simulink library "UAVdesign_net"  (Simulink 7.7)
settings: Solver=ode45  SolverMode=SingleTasking  StartTime=0.0  StopTime=10.0  RelTol=1e-3
undefined symbols (not defined in the file or in its folder): alpha_IERA_IELA_IELA, R_IERA_RA_RA
libraries: UAVdesign_net x75, simulink x13
(part 1 of 8)
settings Model: Creator=Emanuel  LastModifiedBy=Emanuel

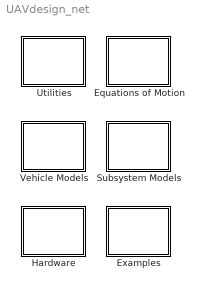
== system UAVdesign_net ==
  Equations of Motion : Subsystem
      mask Display: disp('Equations of\nMotion')
  Examples : Subsystem
      settings: OpenFcn=UAVdesign_net_examples
      mask Display: disp('Examples')
  Hardware : Subsystem
      mask Display: disp('Hardware\nI/O')
  Subsystem Models : Subsystem
      mask Display: disp('Subsystem\nModels')
  Utilities : Subsystem
      mask Display: disp('Utilities')
  Vehicle Models : Subsystem
      mask Display: disp('Vehicle\nModels')

== system UAVdesign_net/Equations of Motion ==
  6DoF Equations of Motion : Subsystem  TreatAsAtomicUnit=on  mask(6DoFEoM){}
      mask help: 6DoF using Euler angles.
      mask Display:
      | port_label('input',1,'V_b(xyz)','texmode','on');
      | port_label('input',2,'\omega_b(xyz)','texmode','on');
      | port_label('input',3,'R_e(NED)','texmode','on');
      | port_label('input',4,'\alpha_e(\phi,\theta,\psi)','texmode','on');
      | port_label('input',5,'F_{ext}(xyz)','texmode','on');
      | port_label('input',6,'M_{ext}(xyz)','texmode','on');
      | port_label('input',7,'m','texmode','on');
      | port_label('input',8,'In_b','texmode','on');
      | port_label('output',1,'V_bdot(xyz)','texmode','on');
      | port_label('output',2,'\omega_bdot(xyz)','texmode','on');
      | port_label('output',3,'R_edot(NED)','texmode','on');
      | port_label('output',4,'\alpha_edot(\phi,\theta,\psi)','texmode','on');
  6DoF Equations of Motion (Quaternions) : Subsystem  TreatAsAtomicUnit=on  mask(6DoFEoMQuaternions){}
      mask help: 6DoF using quaternions.
      mask Display:
      | port_label('input',1,'V_b (xyz)','texmode','on');
      | port_label('input',2,'\omega_b (xyz)','texmode','on');
      | port_label('input',3,'R_e (NED)','texmode','on');
      | port_label('input',4,'q (a_0 a)','texmode','on');
      | port_label('input',5,'F_{ext} (xyz)','texmode','on');
      | port_label('input',6,'M_{ext} (xyz)','texmode','on');
      | port_label('input',7,'m','texmode','on');
      | port_label('input',8,'In_b','texmode','on');
      | port_label('output',1,'V_b^\bullet (xyz)','texmode','on');
      | port_label('output',2,'\omega_b^\bullet (xyz)','texmode','on');
      | port_label('output',3,'R_e^\bullet (NED)','texmode','on');
      | port_label('output',4,'q^\bullet (a_0 a)','texmode','on');

== system UAVdesign_net/Examples ==

== system UAVdesign_net/Hardware ==
  Generic Comm : Subsystem  mask(GenericComm){devicetype=UDP port, com_port='COM4', baud=115200, host_name='192.168.1.10', remote_port=60500, local_port=60500, timeout=1, rx_size=54, handshake=on, sample_time=-1}
      mask prompts: devicetype "Device Type"; com_port "COM port (string between single quotes, e.g. 'COM4' or 'ttyACM0')"; baud "Baud Rate"; host_name "Host Name (string between single quotes, e.g. '192.168.1.10')"; remote_port "Transmit to UDP port"; local_port "Listen on UDP port"; timeout "Timeout (sec)"; rx_size "RX vector size (bytes)"; handshake "Enable handshaking (for the Basestation)"; sample_time "Sample Time"
      mask help:
      | Generic communication block.
      | Allows communication to take place using either a serial port or UDP packets.
      mask init:
      | UAVdesign_net_generic_comm_callback(gcb, 0, 0, com_port, host_name, remote_port, local_port)
      mask StyleString: popup(COM port|UDP port),edit,edit,edit,edit,edit,edit,edit,checkbox,edit
      mask CallbackString: UAVdesign_net_generic_comm_callback(gcb, 1, 0)|||||||||
      mask Display: text(0.1, 0.7, '192.168.1.10'); text(0.1, 0.3, 'L:60500  R:60500')
  Generic Comm Example : Subsystem  mask(GenericCommExample){devicetype=COM port, com_port='COM4', baud=115200, host_name='192.168.1.10', remote_port=60500, local_port=60500, timeout=1}
      mask prompts: devicetype "Device Type"; com_port "COM port"; baud "Baud Rate"; host_name "Host Name"; remote_port "Remote UDP port"; local_port "Local UDP port"; timeout "Timeout (sec)"
      mask help: Example of how to transfer parameters to a Generic Comm block behind a mask.
      mask init:
      | start = 0;
      | a=get_param([gcb '/Generic Comm'], 'MaskStyles');
      | b=get_param(gcb, 'MaskStyles');
      | b{start+1}=a{1};
      | set_param(gcb, 'MaskStyles', b);
      | 
      | a=get_param(gcb, 'MaskValues');
      | b=get_param([gcb '/Generic Comm'], 'MaskValues');
      | b{1}=a{start+1};
      | set_param([gcb '/Generic Comm'], 'MaskValues', b);
      mask StyleString: popup(COM port|UDP port),edit,edit,edit,edit,edit,edit
      mask CallbackString:
      | start = 0;
      | UAVdesign_net_generic_comm_callback(gcb, 1, start)||||||
  GigE Camera : S-Function  FunctionName=gigecomm  Parameters=host,img_size,format,raw_data,soft_trig,timeout,st  EnableBusSupport=off  mask(GigE_Camera){host='192.168.2.20', img_size=[640 480 1], format=Rgb24, raw_data=off, soft_trig=off, timeout=1, st=1/20}
      mask prompts: host "Remote Host (string between single quotes, e.g. '192.168.1.10')"; img_size "Image size [x y N]"; format "Pixel format"; raw_data "Dump raw data"; soft_trig "Software Trigger"; timeout "Timeout (sec)"; st "Sample Time"
      mask help: GigE camera
      mask StyleString: edit,edit,popup(Mono8|Mono16|Bayer8|Bayer16|Rgb24|Rgb48|Yuv411|Yuv422|Yuv444),checkbox,checkbox,edit,edit
      mask Display:
      | text(0.1, 0.7, host)
      | text(0.1, 0.3, [num2str(img_size(1)) 'x' num2str(img_size(2))])
  Serial Port : S-Function  FunctionName=serialcomm  Parameters=port,baud_rate,timeout,tx_enable,rx_enable,receive,num_packets_overrun,num_packets_received,st  EnableBusSupport=off  mask(SerialPort){port='COM4', baud_rate=115200, timeout=1, tx_enable=on, rx_enable=on, receive=46, num_packets_overrun=off, num_packets_received=off, st=-1}
      mask prompts: port "COM port (string between single quotes, e.g. 'COM4' or 'ttyACM0')"; baud_rate "Baud Rate"; timeout "Timeout (sec)"; tx_enable "Enable TX"; rx_enable "Enable RX"; receive "RX vector size (bytes)"; num_packets_overrun "Leave one packet in the RX buffer if more are received"; num_packets_received "Output the number of packets received"; st "Sample Time"
      mask help: Timeout: If positive, the transfers are blocking for the specified amount, and if no data arrives then an error will be generated. If zero, the available data in the buffer (if any) will be transferred. If negative, blocking transfers will occur and no timeout will be used.
      mask Display: disp(port);
  Simulation Rate : S-Function  FunctionName=simulationrate  Parameters=SimSampleTime  EnableBusSupport=off  mask(SimulationRate){SimSampleTime=1/20}
      mask prompts: SimSampleTime "Simulation Sample Time"
      mask help: Slows down the simulation to a rate close to real-time.
      mask Display: disp('Sim Rate')
  Simulation Time : S-Function  FunctionName=display_time_sfun  Parameters=sample_time  EnableBusSupport=off  mask(DisplayTime){sample_time=-1}
      mask prompts: sample_time "Input Sample Time"
      mask help: This block displays the simulation time in the Matlab workspace for debugging purposes.
      mask Display: port_label('Output', 1, 'Time');
  Thread Priority : S-Function  FunctionName=threadpriority  Parameters=PolicySimWin,PolicyExtWin,PolicySimLinux,PolicyExtLinux,PrioritySimWin,PriorityExtWin,PrioritySimLinux,PriorityExtLinux  EnableBusSupport=off  mask(ThreadPriority){PolicySimWin=Normal, PolicyExtWin=Normal, PolicySimLinux=SCHED_OTHER, PolicyExtLinux=SCHED_OTHER, PrioritySimWin=0, PriorityExtWin=0, PrioritySimLinux=0, PriorityExtLinux=-6}
      mask prompts: PolicySimWin "Thread policy (Windows, Simulation)"; PolicyExtWin "Thread policy (Windows, External)"; PolicySimLinux "Thread policy (Linux, Simulation)"; PolicyExtLinux "Thread policy (Linux, External)"; PrioritySimWin "Thread priority (Windows, Simulation)"; PriorityExtWin "Thread priority (Windows, External)"; PrioritySimLinux "Thread priority (Linux, Simulation)"; PriorityExtLinux "Thread priority (Linux, External)"
      mask help:
      | For Linux, the priorities specify:
      |   - the nice value for the SCHED_OTHER policy
      |     (-20 for maximum priority, 19 for minimum, 0 for default)
      |   - the real-time priority for the other two options
      |     (1 for minimum priority, 98 for maximum priority).
      mask StyleString: popup(Normal|Real Time),popup(Normal|Real Time),popup(SCHED_OTHER|SCHED_FIFO|SCHED_RR),popup(SCHED_OTHER|SCHED_FIFO|SCHED_RR),edit,edit,edit,edit
      mask Display: disp('Priority')
  To Multimedia File : S-Function  FunctionName=tomultimediafile  Parameters=format, file_name, force_rate, frame_rate, sample_time  EnableBusSupport=off  mask(ToMMFile){format=Raw, file_name='test.bin', force_rate=off, frame_rate=25, sample_time=-1}
      mask prompts: format "File Format"; file_name "File Name (between commas, e.g. 'test.avi')"; force_rate "Force a specific frame rate in the header"; frame_rate "Frame Rate (to be included in the file header)"; sample_time "Sample Time"
      mask help: Saves the data to a file in different formats.
      mask init:
      | maskval = get_param(gcb, 'MaskValues');
      | visibility = get_param(gcb, 'MaskVisibilities');
      | if strcmp(maskval{3}, 'on')
      |     visibility{4} = 'on';
      | else
      |     visibility{4} = 'off';
      | end
      | set_param(gcb, 'MaskVisibilities', visibility);
      mask StyleString: popup(Raw|AVI|WAV),edit,checkbox,edit,edit
      mask CallbackString:
      | ||maskval = get_param(gcb, 'MaskValues');
      | visibility = get_param(gcb, 'MaskVisibilities');
      | if strcmp(maskval{3}, 'on')
      |     visibility{4} = 'on';
      | else
      |     visibility{4} = 'off';
      | end
      | set_param(gcb, 'MaskVisibilities', visibility);
      | clear maskval visibility
      | ||
      mask Display: disp(file_name)
  Type Conversion : S-Function  FunctionName=datatypeconv_sfun  Parameters=indim, intype, outdim, outtype, signextend  EnableBusSupport=off  mask(TypeConversion){indim=4, intype=uint8, outdim=1, outtype=unsigned double, signextend=off}
      mask prompts: indim "Input Dimension"; intype "Input Type"; outdim "Output Dimension"; outtype "Output Type"; signextend "Sign Extend the Input"
      mask help: Converts between data types while keeping the binary representation.
      mask init:
      | tstr = {'dbl' 'sgl' 'int8' 'uint8' 'int16' 'uint16' 'int32' 'uint32' 'bool' 'udbl' 'usgl'};
      | dispstr = [tstr{intype} ' \rightarrow ' tstr{outtype}];
      mask StyleString: edit,popup(double|single|int8|uint8|int16|uint16|int32|uint32|boolean),edit,popup(double|single|int8|uint8|int16|uint16|int32|uint32|boolean|unsigned double|unsigned single),checkbox
      mask Display: disp(dispstr, 'texmode', 'on')
  UDP : S-Function  FunctionName=udpcomm  Parameters=host,local_port,remote_port,timeout,tx_enable,rx_enable,receive,num_packets_overrun,num_packets_received,handshake,st  EnableBusSupport=off  mask(UDPPort){host='192.168.2.20', remote_port=60500, local_port=60500, timeout=1, tx_enable=on, rx_enable=on, receive=46, num_packets_overrun=off, num_packets_received=off, handshake=on, st=-1}
      mask prompts: host "Remote Host (string between single quotes, e.g. '192.168.1.10')"; remote_port "Transmit to UDP port"; local_port "Listen on UDP port"; timeout "Timeout (sec)"; tx_enable "Enable TX"; rx_enable "Enable RX"; receive "Receive vector size (bytes)"; num_packets_overrun "Leave one packet in the RX buffer if more are received"; num_packets_received "Output the number of packets received"; handshake "Enable handshaking (for the Basestation)"; st "Sample Time"
      mask help: Timeout: If positive, the transfers are blocking for the specified amount, and if no data arrives then an error will be generated. If zero, the available data in the buffer (if any) will be transferred. If negative, blocking transfers will occur and no timeout will be used.
      mask Display:
      | text(0.1, 0.7, host)
      | text(0.1, 0.3, ['L:' num2str(local_port) '  R:' num2str(remote_port)])

== system UAVdesign_net/Subsystem Models ==
  DC Motor (Electrical) : Subsystem  TreatAsAtomicUnit=on
      mask Type: HelicopterMotor
      mask Description: DC Motor model.
      mask Display:
      | port_label('input', 1, 'Parameters', 'texmode', 'on')
      | port_label('input', 2, 'Voltage', 'texmode', 'on')
      | port_label('input', 3, '\Omega_{rotor-stator}', 'texmode', 'on')
      | 
      | port_label('output', 1, '\tau_{motor}', 'texmode', 'on')
  Fin : Subsystem  TreatAsAtomicUnit=on
      mask Type: HelicopterFinModel
      mask Description: Fin model.
      mask Display:
      | port_label('input', 1, 'Parameters', 'texmode', 'on')
      | port_label('input', 2, 'Environment', 'texmode', 'on')
      | port_label('input', 3, 'R_{IELA-B|B}', 'texmode', 'on')
      | port_label('input', 4, 'T_{IERA-IELA}', 'texmode', 'on')
      | port_label('input', 5, 'V_{B-E|B}', 'texmode', 'on')
      | port_label('input', 6, '\omega_{B-E|B}', 'texmode', 'on')
      | port_label('input', 7, 'V_{W|B}', 'texmode', 'on')
      | port_label('input', 8, '\omega_{W|B}', 'texmode', 'on')
      | 
      | port_label('output', 1, 'FM_{B}', 'texmode', 'on')
      | port_label('output', 2, 'FM_{IELA}', 'texmode', 'on')
      | port_label('output', 3, 'd_{IELA}', 'texmode', 'on')
      | port_label('output', 4, 'V \omega_{A|IELA}', 'texmode', 'on')
  Fuselage : Subsystem  TreatAsAtomicUnit=on
      mask Type: HelicopterFuselageModel
      mask Description: Fuselage model.
      mask Display:
      | port_label('input', 1, 'Parameters', 'texmode', 'on')
      | port_label('input', 2, 'Environment', 'texmode', 'on')
      | port_label('input', 3, 'R_{IELA-B|B}', 'texmode', 'on')
      | port_label('input', 4, 'T_{IERA-IELA}', 'texmode', 'on')
      | port_label('input', 5, 'V_{B-E|B}', 'texmode', 'on')
      | port_label('input', 6, '\omega_{B-E|B}', 'texmode', 'on')
      | port_label('input', 7, 'V_{W|B}', 'texmode', 'on')
      | port_label('input', 8, '\omega_{W|B}', 'texmode', 'on')
      | 
      | port_label('output', 1, 'FM_{B}', 'texmode', 'on')
      | port_label('output', 2, 'FM_{IELA}', 'texmode', 'on')
      | port_label('output', 3, 'd_{IELA}', 'texmode', 'on')
      | port_label('output', 4, 'V \omega_{A|IELA}', 'texmode', 'on')
  Helicopter Parameters : Subsystem  mask(HelicopterParameters){}
      mask help:
      | Parameters for a helicopter.
      | Geometry, rotors, fuselage, fins.
      mask init:
      | set_param(gcb, 'LinkStatus', 'none');
      settings: OpenFcn=gui_HelicopterParameters( 'Block', [get_param(gcb, 'Parent') '/' get_param(gcb, 'Name')]);
      mask Display:
      | port_label('output', 1, 'Parameters')
      | port_label('output', 2, 'Geometry')
  Helicopter Rotor : Subsystem  TreatAsAtomicUnit=on
      mask Type: HelicopterRotorModel
      mask Description: Model of a helicopter rotor
      mask Display:
      | port_label('input', 1, 'Parameters', 'texmode', 'on')
      | port_label('input', 2, 'Environment', 'texmode', 'on')
      | port_label('input', 3, 'R_{IELA-B|B}', 'texmode', 'on')
      | port_label('input', 4, 'T_{IERA-IELA}', 'texmode', 'on')
      | port_label('input', 5, 'V_{B-E|B}', 'texmode', 'on')
      | port_label('input', 6, '\omega_{B-E|B}', 'texmode', 'on')
      | port_label('input', 7, 'V^\bullet_{B-E|B}', 'texmode', 'on')
      | port_label('input', 8, '\omega^\bullet_{B-E|B}', 'texmode', 'on')
      | port_label('input', 9, 'V_{W|B}', 'texmode', 'on')
      | port_label('input', 10, '\omega_{W|B}', 'texmode', 'on')
      | port_label('input', 11, '\Omega_{rotor}', 'texmode', 'on')
      | port_label('input', 12, '\Omega^\bullet_{rotor}', 'texmode', 'on')
      | port_label('input', 13, 'controls_{IERA}', 'texmode', 'on')
      | port_label('input', 14, 'tilt^\bullet_{nac}', 'texmode', 'on')
      | port_label('input', 15, 'flap_{(k-1)|IERA}', 'texmode', 'on')
      | port_label('input', 16, 'd_{k-1|IELA}', 'texmode', 'on')
      | port_label('input', 17, 'bt_{k-1}', 'texmode', 'on')
      | port_label('input', 18, 'eps0_{k-1}', 'texmode', 'on')
      | 
      | port_label('output', 1, 'FM_{B}', 'texmode', 'on')
      | port_label('output', 2, 'FM_{IELA}', 'texmode', 'on')
      | port_label('output', 3, 'flap^\bullet_{IERA}', 'texmode', 'on')
      | port_label('output', 4, 'd_{k|IELA}', 'texmode', 'on')
      | port_label('output', 5, 'bt_{k}', 'texmode', 'on')
      | port_label('output', 6, 'eps0_{k}', 'texmode', 'on')
      | port_label('output', 7, 'flap_{k|IERA}', 'texmode', 'on')
      | port_label('output', 8, 'T Q', 'texmode', 'on')
      | port_label('output', 9, 'V \omega_{A|IELA}', 'texmode', 'on')
  Propeller : Subsystem  TreatAsAtomicUnit=on
      mask Type: HelicopterPropellerModel
      mask Description: Model of a rigid propeller
      mask Display:
      | port_label('input', 1, 'Parameters', 'texmode', 'on')
      | port_label('input', 2, 'Environment', 'texmode', 'on')
      | port_label('input', 3, 'R_{IELA-B|B}', 'texmode', 'on')
      | port_label('input', 4, 'T_{IERA-IELA}', 'texmode', 'on')
      | port_label('input', 5, 'V_{B-E|B}', 'texmode', 'on')
      | port_label('input', 6, '\omega_{B-E|B}', 'texmode', 'on')
      | port_label('input', 7, 'V_{W|B}', 'texmode', 'on')
      | port_label('input', 8, '\omega_{W|B}', 'texmode', 'on')
      | port_label('input', 9, '\Omega_{rotor}', 'texmode', 'on')
      | port_label('input', 10, '\tau_{motor}', 'texmode', 'on')
      | port_label('input', 11, 'pitch', 'texmode', 'on')
      | port_label('input', 12, 'd_{k-1|IELA}', 'texmode', 'on')
      | port_label('input', 13, 'bt_{k-1}', 'texmode', 'on')
      | port_label('input', 14, 'eps0_{k-1}', 'texmode', 'on')
      | 
      | port_label('output', 1, 'FM_{B}', 'texmode', 'on')
      | port_label('output', 2, 'FM_{IELA}', 'texmode', 'on')
      | port_label('output', 3, 'd_{k|IELA}', 'texmode', 'on')
      | port_label('output', 4, 'bt_{k}', 'texmode', 'on')
      | port_label('output', 5, 'eps0_{k}', 'texmode', 'on')
      | port_label('output', 6, 'T Q', 'texmode', 'on')
      | port_label('output', 7, 'V \omega_{A|IELA}', 'texmode', 'on')
  Propeller Rotation Dynamics : Subsystem  TreatAsAtomicUnit=on
      mask Type: HelicopterPropellerRotDynamics
      mask Description: The rotation dynamics for a rigid propeller
      mask Display:
      | port_label('input', 1, 'Parameters', 'texmode', 'on')
      | port_label('input', 2, 'T_{IERA-IELA}', 'texmode', 'on')
      | port_label('input', 3, '\tau_{prop} (Q)', 'texmode', 'on')
      | port_label('input', 4, '\tau_{motor}', 'texmode', 'on')
      | port_label('input', 5, '\omega_{B-E|B}', 'texmode', 'on')
      | port_label('input', 6, '\omega^\bullet_{B-E|B}', 'texmode', 'on')
      | port_label('input', 7, '\Omega_{rotor}', 'texmode', 'on')
      | 
      | port_label('output', 1, '\Omega^\bullet_{rotor}', 'texmode', 'on')
  QuadRotor Parameters : Subsystem  InitFcn=|  mask(HelicopterParameters){}
      | bus_PropellerParameters;    
      | bus_ElectricMotorParameters;
      | bus_GeometryParameters;     
      | bus_FuselageParameters;
      mask help:
      | Parameters for a helicopter.
      | Geometry, rotors, fuselage, fins.
      mask init:
      | set_param(gcb, 'LinkStatus', 'none');
      settings: OpenFcn=gui_QuadRotorParameters( 'Block', [get_param(gcb, 'Parent') '/' get_param(gcb, 'Name')]);
      mask Display:
      | port_label('output', 1, 'Parameters')
      | port_label('output', 2, 'Geometry')
  Wing : Subsystem  TreatAsAtomicUnit=on
      mask Type: HelicopterWingModel
      mask Description: Wing model.
      mask Display:
      | port_label('input', 1, 'Parameters', 'texmode', 'on')
      | port_label('input', 2, 'Environment', 'texmode', 'on')
      | port_label('input', 3, 'R_{IELA-B|B}', 'texmode', 'on')
      | port_label('input', 4, 'T_{IERA-IELA}', 'texmode', 'on')
      | port_label('input', 5, 'V_{B-E|B}', 'texmode', 'on')
      | port_label('input', 6, '\omega_{B-E|B}', 'texmode', 'on')
      | port_label('input', 7, 'V_{W|B}', 'texmode', 'on')
      | port_label('input', 8, '\omega_{W|B}', 'texmode', 'on')
      | 
      | port_label('output', 1, 'FM_{B}', 'texmode', 'on')
      | port_label('output', 2, 'FM_{IELA}', 'texmode', 'on')
      | port_label('output', 3, 'd_{IELA}', 'texmode', 'on')
      | port_label('output', 4, 'V \omega_{A|IELA}', 'texmode', 'on')

== system UAVdesign_net/Utilities ==
  Axes : Subsystem
      mask Display: disp('Axes\nTransf.')
  Continuous : Subsystem
      mask Display: disp('Continuous')
  Kalman Filter : Subsystem
      mask Display: disp('Kalman\nFilter')
  Math : Subsystem
      mask Display: disp('Math\nOperations')
  Numeric Perturbation : Subsystem
      mask Display: disp('Numeric\nPerturbation')
  Unit Conversion : Subsystem
      mask Display: disp('Unit\nConversions')

== system UAVdesign_net/Vehicle Models ==
  Helicopter Model : Subsystem  InitFcn=|  TreatAsAtomicUnit=on
      | bus_RotorParameters;
      | bus_FuselageParameters;
      | bus_FinParameters;
      | bus_GeometryParameters;
      | bus_Environment;
      mask Type: HelicopterModel
      mask Description:
      | Model of a helicopter.
      | Derived from "Introduction to Helicopter and Tiltrotor Flight Simulation" by Mark Dreier.
      mask Display:
      | port_label('input', 1, 'Parameters (bus)', 'texmode', 'on')
      | port_label('input', 2, 'Geometry (bus)', 'texmode', 'on')
      | port_label('input', 3, 'Environment (bus)', 'texmode', 'on')
      | port_label('input', 4, 'controls', 'texmode', 'on')
      | port_label('input', 5, '\Omega_{rotor} MR', 'texmode', 'on')
      | port_label('input', 6, '\Omega_{rotor} TR', 'texmode', 'on')
      | port_label('input', 7, 'xc', 'texmode', 'on')
      | port_label('input', 8, 'xc^\bullet_{k-1}', 'texmode', 'on')
      | port_label('input', 9, 'xd_{k-1}', 'texmode', 'on')
      | 
      | port_label('output', 1, 'xc^\bullet', 'texmode', 'on')
      | port_label('output', 2, 'xd_{k}', 'texmode', 'on')
      | port_label('output', 3, 'flap_{k}', 'texmode', 'on')
      | port_label('output', 4, '[info] FM_{CG}', 'texmode', 'on')
      | port_label('output', 5, '[info] FM_{IELA}', 'texmode', 'on')
      | port_label('output', 6, '[info] d_{IELA}', 'texmode', 'on')
      | port_label('output', 7, '[info] V \omega_{W|IELA}', 'texmode', 'on')
      | port_label('output', 8, '[info] V \omega_{A|IELA}', 'texmode', 'on')
      | port_label('output', 9, '[info] TQ rotors', 'texmode', 'on')
  Helicopter Parameters : Subsystem  mask(HelicopterParameters){}
      mask help:
      | Parameters for a helicopter.
      | Geometry, rotors, fuselage, fins.
      mask init:
      | set_param(gcb, 'LinkStatus', 'none');
      settings: OpenFcn=gui_HelicopterParameters( 'Block', [get_param(gcb, 'Parent') '/' get_param(gcb, 'Name')]);
      mask Display:
      | port_label('output', 1, 'Parameters')
      | port_label('output', 2, 'Geometry')
  Quad-Rotor Model (Momentum) : Subsystem  InitFcn=|  TreatAsAtomicUnit=on
      | bus_PropellerParameters;    
      | bus_ElectricMotorParameters;
      | bus_FuselageParameters;     
      | bus_GeometryParameters;     
      | bus_Environment;
      mask Type: HelicopterModel
      mask Description: Model of a quadrotor
      mask Display:
      | port_label('input', 1, 'Parameters (bus)', 'texmode', 'on')
      | port_label('input', 2, 'Geometry (bus)', 'texmode', 'on')
      | port_label('input', 3, 'Environment (bus)', 'texmode', 'on')
      | port_label('input', 4, 'V_{mot}', 'texmode', 'on')
      | port_label('input', 5, 'Wind_e', 'texmode', 'on')
      | port_label('input', 6, 'xc', 'texmode', 'on')
      | port_label('input', 7, 'xd_{k-1}', 'texmode', 'on')
      | 
      | port_label('output', 1, 'info (bus)', 'texmode', 'on')
      | port_label('output', 2, 'xc^\bullet', 'texmode', 'on')
      | port_label('output', 3, 'xd_{k}', 'texmode', 'on')
  QuadRotor Parameters : Subsystem  InitFcn=|  mask(HelicopterParameters){}
      | bus_PropellerParameters;    
      | bus_ElectricMotorParameters;
      | bus_GeometryParameters;     
      | bus_FuselageParameters;
      mask help:
      | Parameters for a helicopter.
      | Geometry, rotors, fuselage, fins.
      mask init:
      | set_param(gcb, 'LinkStatus', 'none');
      settings: OpenFcn=gui_QuadRotorParameters( 'Block', [get_param(gcb, 'Parent') '/' get_param(gcb, 'Name')]);
      mask Display:
      | port_label('output', 1, 'Parameters')
      | port_label('output', 2, 'Geometry')
  wires:
  QuadRotor Parameters/1(Parameters) -> Quad-Rotor Model (Momentum)/1(ParametersBus)
  QuadRotor Parameters/2(Geometry) -> Quad-Rotor Model (Momentum)/2(GeometryBus)
  Helicopter Parameters/1(Parameters) -> Helicopter Model/1(ParametersBus)
  Helicopter Parameters/2(Geometry) -> Helicopter Model/2(GeometryBus)

== system UAVdesign_net/Equations of Motion/6DoF Equations of Motion ==
  Body velocities (V_b) : Inport  PortDimensions=3
  Angular velocities (omega_b) : Inport  Port=2  PortDimensions=3
  Inertial positions (R_e) : Inport  Port=3  PortDimensions=3
  Euler angles(Alpha_e) : Inport  Port=4  PortDimensions=3
  Forces (F_xyz) : Inport  Port=5  PortDimensions=3
  Moments (M_xyz) : Inport  Port=6  PortDimensions=3
  Mass (m) : Inport  Port=7  PortDimensions=1
  Inertia matrix (In_b) : Inport  Port=8  PortDimensions=[3 3]
  3x3 Cross Product : UAVdesign_net/Utilities/Math/3x3 Cross Product  SystemSampleTime=-1
  3x3 Cross Product1 : UAVdesign_net/Utilities/Math/3x3 Cross Product  SystemSampleTime=-1
  Euler Rotation Matrix from Body to Earth : UAVdesign_net/Utilities/Axes/Euler Rotation Matrix from Body to Earth  SystemSampleTime=-1
  Invert  3x3 Matrix1 : UAVdesign_net/Utilities/Math/Invert  3x3 Matrix  SystemSampleTime=-1
  Math Function : Math  Operator=reciprocal  SaturateOnIntegerOverflow=on
  Product{,1,4..5} (4 alike) : Product  Multiplication=Matrix(*)  RndMeth=Zero
  Product2 : Product  RndMeth=Zero
  Product3 : Product  RndMeth=Zero
  Rotation Matrix for angular rates Body to Earth : UAVdesign_net/Utilities/Axes/Rotation Matrix for angular rates Body to Earth  SystemSampleTime=-1
  Sum : Sum  Inputs=|+-
  Sum1 : Sum  Inputs=|+-
  Terminator : Terminator
  Body accelerations (V_b_dot) : Outport
  Angular accelerations (omega_b_dot) : Outport  Port=2
  Inertial velocities (R_e_dot) : Outport  Port=3
  Euler velocities (alpha_e_dot) : Outport  Port=4
  wires:
  Rotation Matrix for angular rates Body to Earth/1 -> Product1/1
  Inertial positions (R_e)/1 -> Terminator/1
  Product4/1 -> Angular accelerations (omega_b_dot)/1
  Product5/1 -> 3x3 Cross Product1/2
  3x3 Cross Product1/1 -> Sum1/2
  Moments (M_xyz)/1 -> Sum1/1
  Sum1/1 -> Product4/2
  Invert  3x3 Matrix1/1 -> Product4/1
  Inertia matrix (In_b)/1 -> Invert  3x3 Matrix1/1, Product5/1
  Product2/1 -> Body accelerations (V_b_dot)/1
  Product3/1 -> 3x3 Cross Product/2
  3x3 Cross Product/1 -> Sum/2
  Forces (F_xyz)/1 -> Sum/1
  Sum/1 -> Product2/2
  Math Function/1 -> Product2/1
  Mass (m)/1 -> Math Function/1, Product3/1
  Product1/1 -> Euler velocities (alpha_e_dot)/1
  Angular velocities (omega_b)/1 -> 3x3 Cross Product/1, 3x3 Cross Product1/1, Product5/2, Product1/2
  Product/1 -> Inertial velocities (R_e_dot)/1
  Body velocities (V_b)/1 -> Product3/2, Product/2
  Euler Rotation Matrix from Body to Earth/1 -> Product/1
  Euler angles(Alpha_e)/1 -> Rotation Matrix for angular rates Body to Earth/1, Euler Rotation Matrix from Body to Earth/1

== system UAVdesign_net/Equations of Motion/6DoF Equations of Motion (Quaternions) ==
  V_b : Inport  PortDimensions=3
  omega_b : Inport  Port=2  PortDimensions=3
  R_e : Inport  Port=3  PortDimensions=3
  q : Inport  Port=4  PortDimensions=4
  F_xyz : Inport  Port=5  PortDimensions=3
  M_xyz : Inport  Port=6  PortDimensions=3
  Mass : Inport  Port=7  PortDimensions=1
  Inertia matrix (In_b) : Inport  Port=8  PortDimensions=[3 3]
  3x3 Cross Product : UAVdesign_net/Utilities/Math/3x3 Cross Product  SystemSampleTime=-1
  3x3 Cross Product1 : UAVdesign_net/Utilities/Math/3x3 Cross Product  SystemSampleTime=-1
  Divide : Product  Inputs=*/
  Gain : Gain  Gain=1/2
  Invert  3x3 Matrix : UAVdesign_net/Utilities/Math/Invert  3x3 Matrix  SystemSampleTime=-1
  Product : Product  Multiplication=Matrix(*)  RndMeth=Zero
  Product1 : Product  Multiplication=Matrix(*)  RndMeth=Zero
  Quaternion Multiplication : UAVdesign_net/Utilities/Math/Quaternion Multiplication  SystemSampleTime=-1
  Quaternion Rotation (E<B) : UAVdesign_net/Utilities/Math/Quaternion Rotation (E<B)  SystemSampleTime=-1
  Sum : Sum  Inputs=|-+
  Sum1 : Sum  Inputs=+-|
  Terminator : Terminator
  Vector to Quaternion : UAVdesign_net/Utilities/Math/Vector to Quaternion  SystemSampleTime=-1
  V_b_dot : Outport
  omega_b_dot : Outport  Port=2
  R_e_dot : Outport  Port=3
  q_dot : Outport  Port=4
  wires:
  Quaternion Multiplication/1 -> q_dot/1
  Vector to Quaternion/1 -> Quaternion Multiplication/2
  Gain/1 -> Quaternion Multiplication/1
  R_e/1 -> Terminator/1
  Quaternion Rotation (E<B)/1 -> R_e_dot/1
  q/1 -> Gain/1, Quaternion Rotation (E<B)/1
  Product/1 -> omega_b_dot/1
  3x3 Cross Product1/1 -> Sum1/2
  M_xyz/1 -> Sum1/1
  Product1/1 -> 3x3 Cross Product1/2
  Invert  3x3 Matrix/1 -> Product/1
  Sum1/1 -> Product/2
  Inertia matrix (In_b)/1 -> Product1/1, Invert  3x3 Matrix/1
  Sum/1 -> V_b_dot/1
  Divide/1 -> Sum/2
  3x3 Cross Product/1 -> Sum/1
  V_b/1 -> Quaternion Rotation (E<B)/2, 3x3 Cross Product/2
  omega_b/1 -> Vector to Quaternion/1, Product1/2, 3x3 Cross Product1/1, 3x3 Cross Product/1
  Mass/1 -> Divide/2
  F_xyz/1 -> Divide/1

== system UAVdesign_net/Hardware/Generic Comm ==
  TX : Inport
  UDP : UAVdesign_net/Hardware/UDP  host=host_name  remote_port=remote_port  local_port=local_port  timeout=timeout  tx_enable=on  rx_enable=on  receive=rx_size  num_packets_overrun=off  num_packets_received=on  handshake=on  st=sample_time
  RX : Outport
  num_rx_packets : Outport  Port=2
  wires:
  TX/1 -> UDP/1
  UDP/1 -> RX/1
  UDP/2 -> num_rx_packets/1

== system UAVdesign_net/Hardware/Generic Comm Example ==
  In1 : Inport
  Generic Comm : UAVdesign_net/Hardware/Generic Comm  SystemSampleTime=-1  devicetype=COM port  com_port=com_port  baud=baud  host_name=host_name  remote_port=remote_port  local_port=local_port  timeout=timeout  rx_size=54  handshake=on  sample_time=-1
  Out1 : Outport
  Out2 : Outport  Port=2

== system UAVdesign_net/Subsystem Models/DC Motor (Electrical) ==
  Parameters : Inport
  V : Inport  Port=2  PortDimensions=1
  omega : Inport  Port=3  PortDimensions=1
  Bus Selector : BusSelector  OutputSignals=R,Kv,Kt
  Divide : Product  Inputs=*/
  Product : Product  RndMeth=Zero
  Product1 : Product  Inputs=**/  RndMeth=Zero
  Sum : Sum  Inputs=|+-
  tork : Outport  PortDimensions=1
  wires:
  Parameters/1 -> Bus Selector/1
  Bus Selector/1 -> Divide/2  "<R>"
  Bus Selector/2 -> Product1/3  "<Kv>"
  Bus Selector/3 -> Product/1, Product1/1  "<Kt>"
  V/1 -> Product/2
  Product/1 -> Sum/1
  Product1/1 -> Sum/2
  Sum/1 -> Divide/1
  Divide/1 -> tork/1
  omega/1 -> Product1/2

== system UAVdesign_net/Subsystem Models/Fin ==
  Parameters : Inport  OutDataTypeStr=Bus: FinParameters
  Environment : Inport  Port=2  OutDataTypeStr=Bus: Environment
  R_IELA_B_B : Inport  Port=3  PortDimensions=3
  T_IERA_IELA : Inport  Port=4  PortDimensions=[3 3]
  V_B_E_B : Inport  Port=5  PortDimensions=3
  omega_B_E_B : Inport  Port=6  PortDimensions=3
  V_W : Inport  Port=7  PortDimensions=3
  omega_W : Inport  Port=8  PortDimensions=3
  CG to IELA : Subsystem
      mask Display:
      | port_label('input', 1, 'R_{IELA-B|B}', 'texmode', 'on')
      | port_label('input', 2, 'V_{B-E|B}', 'texmode', 'on')
      | port_label('input', 3, '\omega_{B-E|B}', 'texmode', 'on')
      | port_label('output', 1, 'V_{IELA-E|IELA}', 'texmode', 'on')
      | port_label('output', 2, '\omega_{IELA-E|IELA}', 'texmode', 'on')
  Fin Model (IERA) : Subsystem
      mask Display:
      | port_label('input', 1, 'Parameters', 'texmode', 'on')
      | port_label('input', 2, 'Environment', 'texmode', 'on')
      | port_label('input', 3, 'V_{A}', 'texmode', 'on')
      | port_label('input', 4, '\omega_{A}', 'texmode', 'on')
      | port_label('input', 5, 'V_{W}', 'texmode', 'on')
      | port_label('input', 6, '\omega_{W}', 'texmode', 'on')
      | port_label('input', 7, 'control', 'texmode', 'on')
      | 
      | port_label('output', 1, 'FM_{I}', 'texmode', 'on')
      | port_label('output', 2, 'FM_{A}', 'texmode', 'on')
      | port_label('output', 3, 'd_{k}', 'texmode', 'on')
  IELA to CG : Subsystem
      mask Display:
      | port_label('input', 1, 'R_{IELA-B|B}', 'texmode', 'on')
      | port_label('input', 2, 'FM_{IELA}', 'texmode', 'on')
      | port_label('output', 1, 'FM_{B}', 'texmode', 'on')
  IELA to IERA : Subsystem
      mask Display:
      | port_label('input', 1, 'T_{IERA-IELA}', 'texmode', 'on')
      | port_label('input', 2, 'V_{A|IELA}', 'texmode', 'on')
      | port_label('input', 3, '\omega_{A|IELA}', 'texmode', 'on')
      | port_label('input', 4, 'V_{W|IELA}', 'texmode', 'on')
      | port_label('input', 5, '\omega_{W|IELA}', 'texmode', 'on')
      | 
      | port_label('output', 1, 'V_{A|IERA}', 'texmode', 'on')
      | port_label('output', 2, '\omega_{A|IERA}', 'texmode', 'on')
      | port_label('output', 3, 'V_{W|IERA}', 'texmode', 'on')
      | port_label('output', 4, '\omega_{W|IERA}', 'texmode', 'on')
  IERA to IELA : Subsystem
      mask Display:
      | port_label('input', 1, 'T_{IELA-IERA}', 'texmode', 'on')
      | port_label('input', 2, 'FM_{I|IERA}', 'texmode', 'on')
      | port_label('input', 3, 'FM_{A|IERA}', 'texmode', 'on')
      | port_label('input', 4, 'd_{IERA}', 'texmode', 'on')
      | port_label('output', 1, 'FM_{I|IELA}', 'texmode', 'on')
      | port_label('output', 2, 'FM_{A|IELA}', 'texmode', 'on')
      | port_label('output', 3, 'd_{IELA}', 'texmode', 'on')
  No control : Constant  Value=0
  Sum : Sum  Inputs=++|
  Sum3 : Sum  Inputs=|+-
  Sum4 : Sum  Inputs=|+-
  Transpose : Subsystem
      mask Display: disp('A^T', 'texmode', 'on')
  Vector Concatenate : Concatenate  Mode=Vector
  FM_B : Outport  PortDimensions=6
  FM_IELA : Outport  Port=2  PortDimensions=6
  d (k) : Outport  Port=3  PortDimensions=3
  V_om_A : Outport  Port=4  PortDimensions=6
  wires:
  IERA to IELA/1(FM_I_IELA) -> Sum/1
  Sum/1 -> IELA to CG/2(FM_IELA), FM_IELA/1
  Fin Model (IERA)/2(FM_A) -> IERA to IELA/3(FM_A_IERA)
  Fin Model (IERA)/1(FM_I) -> IERA to IELA/2(FM_I_IERA)
  omega_B_E_B/1 -> CG to IELA/3(omega_B_E|B)
  IELA to IERA/1(V_A_IERA) -> Fin Model (IERA)/3(V_A)
  IELA to IERA/2(omega_A_IERA) -> Fin Model (IERA)/4(omega_A)
  IELA to IERA/3(V_W_IERA) -> Fin Model (IERA)/5(V_W)
  IELA to IERA/4(omega_W_IERA) -> Fin Model (IERA)/6(omega_W)
  IERA to IELA/2(FM_A_IELA) -> Sum/2
  Fin Model (IERA)/3(d (k)) -> IERA to IELA/4(d_IERA)
  Parameters/1 -> Fin Model (IERA)/1(Parameters)
  Environment/1 -> Fin Model (IERA)/2(Environment)
  T_IERA_IELA/1 -> IELA to IERA/1(T_IERA_IELA), Transpose/1(In)
  V_B_E_B/1 -> CG to IELA/2(V_B-E|B)
  Transpose/1(Out) -> IERA to IELA/1(T_IELA_IERA)
  IELA to CG/1(FM_B) -> FM_B/1
  IERA to IELA/3(d_IELA) -> d (k)/1
  R_IELA_B_B/1 -> CG to IELA/1(R_IELA-B|B), IELA to CG/1(R_IELA_B_B)
  CG to IELA/1(V_IELA-E|IELA) -> Sum3/1
  Sum3/1 -> IELA to IERA/2(V_A_IELA), Vector Concatenate/1
  CG to IELA/2(omega_IELA-E|IELA) -> Sum4/1
  Sum4/1 -> IELA to IERA/3(omega_A_IELA), Vector Concatenate/2
  V_W/1 -> Sum3/2, IELA to IERA/4(V_W_IELA)
  omega_W/1 -> Sum4/2, IELA to IERA/5(omega_W_IELA)
  No control/1 -> Fin Model (IERA)/7(control)
  Vector Concatenate/1 -> V_om_A/1

== system UAVdesign_net/Subsystem Models/Fuselage ==
  Parameters : Inport  OutDataTypeStr=Bus: FuselageParameters
  Environment : Inport  Port=2  OutDataTypeStr=Bus: Environment
  R_IELA_B_B : Inport  Port=3  PortDimensions=3
  T_IERA_IELA : Inport  Port=4  PortDimensions=[3 3]
  V_B_E_B : Inport  Port=5  PortDimensions=3
  omega_B_E_B : Inport  Port=6  PortDimensions=3
  V_W : Inport  Port=7  PortDimensions=3
  omega_W : Inport  Port=8  PortDimensions=3
  CG to IELA : Subsystem
      mask Display:
      | port_label('input', 1, 'R_{IELA-B|B}', 'texmode', 'on')
      | port_label('input', 2, 'V_{B-E|B}', 'texmode', 'on')
      | port_label('input', 3, '\omega_{B-E|B}', 'texmode', 'on')
      | port_label('output', 1, 'V_{IELA-E|IELA}', 'texmode', 'on')
      | port_label('output', 2, '\omega_{IELA-E|IELA}', 'texmode', 'on')
  Fuselage Model (IERA) : Subsystem
      mask Display:
      | port_label('input', 1, 'Parameters', 'texmode', 'on')
      | port_label('input', 2, 'Environment', 'texmode', 'on')
      | port_label('input', 3, 'V_{A}', 'texmode', 'on')
      | port_label('input', 4, '\omega_{A}', 'texmode', 'on')
      | port_label('input', 5, 'V_{W}', 'texmode', 'on')
      | port_label('input', 6, '\omega_{W}', 'texmode', 'on')
      | 
      | port_label('output', 1, 'FM_{I}', 'texmode', 'on')
      | port_label('output', 2, 'FM_{A}', 'texmode', 'on')
      | port_label('output', 3, 'd_{k}', 'texmode', 'on')
  IELA to CG : Subsystem
      mask Display:
      | port_label('input', 1, 'R_{IELA-B|B}', 'texmode', 'on')
      | port_label('input', 2, 'FM_{IELA}', 'texmode', 'on')
      | port_label('output', 1, 'FM_{B}', 'texmode', 'on')
  IELA to IERA : Subsystem
      mask Display:
      | port_label('input', 1, 'T_{IERA-IELA}', 'texmode', 'on')
      | port_label('input', 2, 'V_{A|IELA}', 'texmode', 'on')
      | port_label('input', 3, '\omega_{A|IELA}', 'texmode', 'on')
      | port_label('input', 4, 'V_{W|IELA}', 'texmode', 'on')
      | port_label('input', 5, '\omega_{W|IELA}', 'texmode', 'on')
      | 
      | port_label('output', 1, 'V_{A|IERA}', 'texmode', 'on')
      | port_label('output', 2, '\omega_{A|IERA}', 'texmode', 'on')
      | port_label('output', 3, 'V_{W|IERA}', 'texmode', 'on')
      | port_label('output', 4, '\omega_{W|IERA}', 'texmode', 'on')
  IERA to IELA : Subsystem
      mask Display:
      | port_label('input', 1, 'T_{IELA-IERA}', 'texmode', 'on')
      | port_label('input', 2, 'FM_{I|IERA}', 'texmode', 'on')
      | port_label('input', 3, 'FM_{A|IERA}', 'texmode', 'on')
      | port_label('input', 4, 'd_{IERA}', 'texmode', 'on')
      | port_label('output', 1, 'FM_{I|IELA}', 'texmode', 'on')
      | port_label('output', 2, 'FM_{A|IELA}', 'texmode', 'on')
      | port_label('output', 3, 'd_{IELA}', 'texmode', 'on')
  Sum : Sum  Inputs=++|
  Sum3 : Sum  Inputs=|+-
  Sum4 : Sum  Inputs=|+-
  Transpose : Subsystem
      mask Display: disp('A^T', 'texmode', 'on')
  Vector Concatenate : Concatenate  Mode=Vector
  FM_B : Outport  PortDimensions=6
  FM_IELA : Outport  Port=2  PortDimensions=6
  d (k) : Outport  Port=3  PortDimensions=3
  V_om_A : Outport  Port=4  PortDimensions=6
  wires:
  IERA to IELA/1(FM_I_IELA) -> Sum/1
  Sum/1 -> IELA to CG/2(FM_IELA), FM_IELA/1
  Fuselage Model (IERA)/2(FM_A) -> IERA to IELA/3(FM_A_IERA)
  Fuselage Model (IERA)/1(FM_I) -> IERA to IELA/2(FM_I_IERA)
  omega_B_E_B/1 -> CG to IELA/3(omega_B_E|B)
  IELA to IERA/1(V_A_IERA) -> Fuselage Model (IERA)/3(V_A)
  IELA to IERA/2(omega_A_IERA) -> Fuselage Model (IERA)/4(omega_A)
  IELA to IERA/3(V_W_IERA) -> Fuselage Model (IERA)/5(V_W)
  IELA to IERA/4(omega_W_IERA) -> Fuselage Model (IERA)/6(omega_W)
  IERA to IELA/2(FM_A_IELA) -> Sum/2
  Fuselage Model (IERA)/3(d (k)) -> IERA to IELA/4(d_IERA)
  Parameters/1 -> Fuselage Model (IERA)/1(Parameters)
  Environment/1 -> Fuselage Model (IERA)/2(Environment)
  T_IERA_IELA/1 -> IELA to IERA/1(T_IERA_IELA), Transpose/1(In)
  V_B_E_B/1 -> CG to IELA/2(V_B-E|B)
  Transpose/1(Out) -> IERA to IELA/1(T_IELA_IERA)
  IELA to CG/1(FM_B) -> FM_B/1
  IERA to IELA/3(d_IELA) -> d (k)/1
  R_IELA_B_B/1 -> CG to IELA/1(R_IELA-B|B), IELA to CG/1(R_IELA_B_B)
  CG to IELA/1(V_IELA-E|IELA) -> Sum3/1
  Sum3/1 -> IELA to IERA/2(V_A_IELA), Vector Concatenate/1
  CG to IELA/2(omega_IELA-E|IELA) -> Sum4/1
  Sum4/1 -> IELA to IERA/3(omega_A_IELA), Vector Concatenate/2
  V_W/1 -> Sum3/2, IELA to IERA/4(V_W_IELA)
  omega_W/1 -> Sum4/2, IELA to IERA/5(omega_W_IELA)
  Vector Concatenate/1 -> V_om_A/1

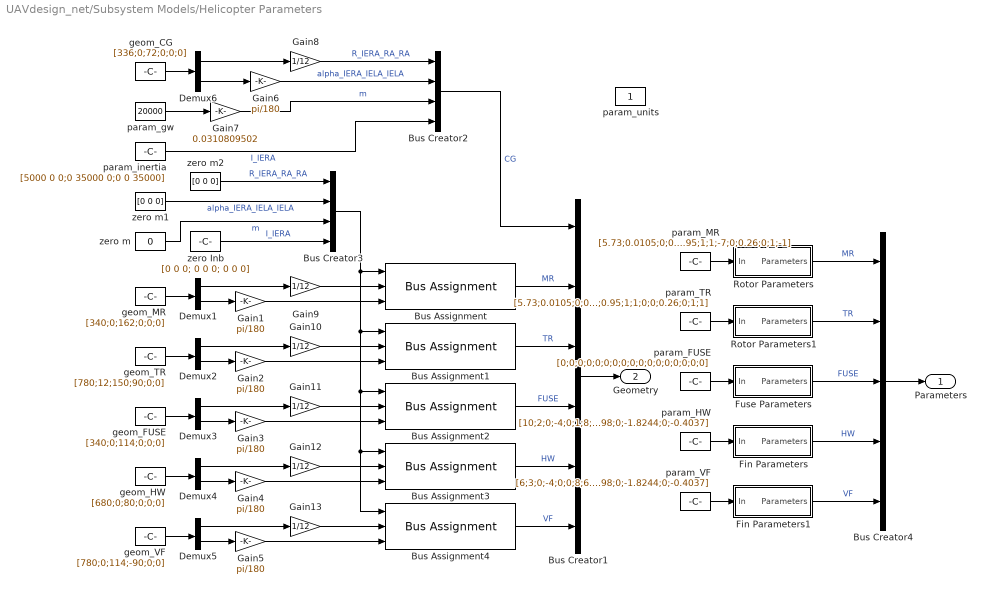
== system UAVdesign_net/Subsystem Models/Helicopter Parameters ==
  Bus Assignment{,1..4} (5 alike) : BusAssignment  AssignedSignals=R_IERA_RA_RA,alpha_IERA_IELA_IELA
  Bus Creator1 : BusCreator  Inputs=6
  Bus Creator2 : BusCreator  OutDataTypeStr=Bus: GeometryParameters
  Bus Creator3 : BusCreator  OutDataTypeStr=Bus: GeometryParameters
  Bus Creator4 : BusCreator  Inputs=5
  Demux{1..6} (6 alike) : Demux  Outputs=2
  Fin Parameters : Subsystem
  Fin Parameters1 : Subsystem
  Fuse Parameters : Subsystem
  Gain{1..6} (6 alike) : Gain  Gain=pi/180
  Gain{8..13} (6 alike) : Gain  Gain=1/12
  Gain7 : Gain  Gain=0.0310809502
  Rotor Parameters : Subsystem
  Rotor Parameters1 : Subsystem
  geom_CG : Constant  Value=[336;0;72;0;0;0]
  geom_FUSE : Constant  Value=[340;0;114;0;0;0]
  geom_HW : Constant  Value=[680;0;80;0;0;0]
  geom_MR : Constant  Value=[340;0;162;0;0;0]
  geom_TR : Constant  Value=[780;12;150;90;0;0]
  geom_VF : Constant  Value=[780;0;114;-90;0;0]
  param_FUSE : Constant  Value=[0;0;0;0;0;0;0;0;0;0;0;0;0;0;0;0;0]
  param_HW : Constant  Value=[10;2;0;-4;0;1;8;6.13;0.9682;1.8898;0;-1.8244;0;-0.4037]
  param_MR : Constant  Value=[5.73;0.0105;0;0.01325;0;-15;0;0;7;30;2.5;0.95;1;1;-7;0;0.26;0;1;-1]
  param_TR : Constant  Value=[5.73;0.0105;0;0.01325;0;-45;0;0;4;6.5;1.25;0.95;1;1;0;0;0.26;0;1;1]
  param_VF : Constant  Value=[6;3;0;-4;0;0;8;6.1311;0.9682;1.8898;0;-1.8244;0;-0.4037]
  param_gw : Constant  Value=20000
  param_inertia : Constant  Value=[5000 0 0;0 35000 0;0 0 35000]
  param_units : Constant
  zero Inb : Constant  Value=[0 0 0; 0 0 0; 0 0 0]
  zero m : Constant  Value=0
  zero m1 : Constant  Value=[0 0 0]
  zero m2 : Constant  Value=[0 0 0]
  Parameters : Outport
  Geometry : Outport  Port=2
  wires:
  Gain13/1 -> Bus Assignment4/2
  Gain12/1 -> Bus Assignment3/2
  Gain11/1 -> Bus Assignment2/2
  Gain10/1 -> Bus Assignment1/2
  Gain9/1 -> Bus Assignment/2
  Gain8/1 -> Bus Creator2/1  "R_IERA_RA_RA"
  Gain7/1 -> Bus Creator2/3  "m"
  Gain6/1 -> Bus Creator2/2  "alpha_IERA_IELA_IELA"
  Gain5/1 -> Bus Assignment4/3
  Gain4/1 -> Bus Assignment3/3
  Gain3/1 -> Bus Assignment2/3
  Gain2/1 -> Bus Assignment1/3
  Gain1/1 -> Bus Assignment/3
  param_HW/1 -> Fin Parameters/1(In)
  Fin Parameters/1(Parameters) -> Bus Creator4/4  "HW"
  Fin Parameters1/1(Parameters) -> Bus Creator4/5  "VF"
  param_VF/1 -> Fin Parameters1/1(In)
  Fuse Parameters/1(Parameters) -> Bus Creator4/3  "FUSE"
  param_FUSE/1 -> Fuse Parameters/1(In)
  param_TR/1 -> Rotor Parameters1/1(In)
  Rotor Parameters1/1(Parameters) -> Bus Creator4/2  "TR"
  param_MR/1 -> Rotor Parameters/1(In)
  Rotor Parameters/1(Parameters) -> Bus Creator4/1  "MR"
  Bus Creator4/1 -> Parameters/1
  zero m2/1 -> Bus Creator3/1  "R_IERA_RA_RA"
  zero Inb/1 -> Bus Creator3/4  "I_IERA"
  zero m1/1 -> Bus Creator3/2  "alpha_IERA_IELA_IELA"
  zero m/1 -> Bus Creator3/3  "m"
  Bus Creator3/1 -> Bus Assignment3/1, Bus Assignment4/1, Bus Assignment2/1, Bus Assignment1/1, Bus Assignment/1
  geom_CG/1 -> Demux6/1
  geom_VF/1 -> Demux5/1
  Demux5/2 -> Gain5/1
  Demux5/1 -> Gain13/1
  geom_HW/1 -> Demux4/1
  Demux4/2 -> Gain4/1
  Demux4/1 -> Gain12/1
  geom_FUSE/1 -> Demux3/1
  Demux3/2 -> Gain3/1
  Demux3/1 -> Gain11/1
  geom_TR/1 -> Demux2/1
  Demux2/2 -> Gain2/1
  Demux2/1 -> Gain10/1
  geom_MR/1 -> Demux1/1
  Demux1/2 -> Gain1/1
  Demux1/1 -> Gain9/1
  Bus Assignment/1 -> Bus Creator1/2  "MR"
  param_inertia/1 -> Bus Creator2/4  "I_IERA"
  param_gw/1 -> Gain7/1
  Demux6/2 -> Gain6/1
  Demux6/1 -> Gain8/1
  Bus Creator1/1 -> Geometry/1
  Bus Assignment4/1 -> Bus Creator1/6  "VF"
  Bus Assignment3/1 -> Bus Creator1/5  "HW"
  Bus Assignment2/1 -> Bus Creator1/4  "FUSE"
  Bus Assignment1/1 -> Bus Creator1/3  "TR"
  Bus Creator2/1 -> Bus Creator1/1  "CG"
